simulink model "Lab1_mdl"  (R2013b)
settings: Solver=ode3  StartTime=0.0  StopTime=100.0  FixedStep=10e-3  RelTol=1e-3
undefined symbols (not defined in the file or in its folder): A, B, C
settings Model: Creator=user  LastModifiedBy=user
settings DataIOCC: LimitDataPoints=off

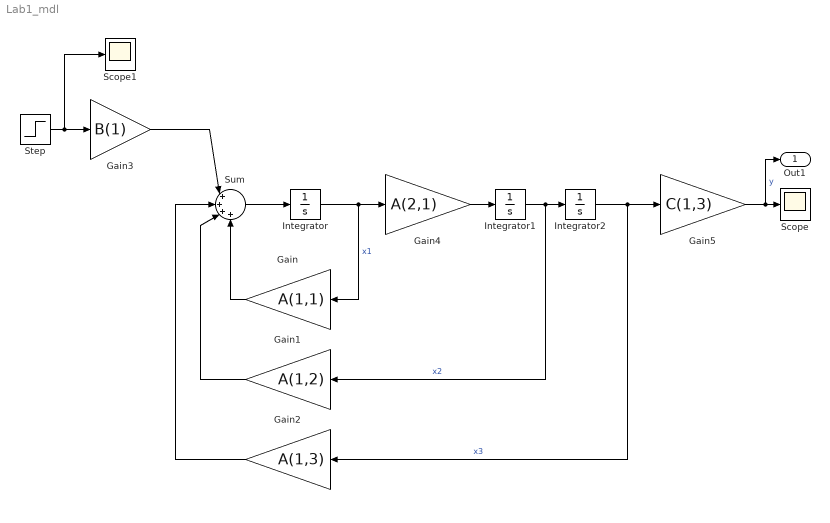
== system Lab1_mdl ==
  Gain : Gain  Gain=A(1,1)
  Gain1 : Gain  Gain=A(1,2)
  Gain2 : Gain  Gain=A(1,3)
  Gain3 : Gain  Gain=B(1)
  Gain4 : Gain  Gain=A(2,1)
  Gain5 : Gain  Gain=C(1,3)
  Integrator : Integrator
  Integrator1 : Integrator
  Integrator2 : Integrator
  Scope : Scope
      settings: SaveName=ContMdl_out
  Scope1 : Scope
      settings: SaveName=SetPoint
  Step : Step  Time=0  SampleTime=0
  Sum : Sum  Inputs=|++++
  Out1 : Outport
  wires:
  Sum/1 -> Integrator/1
  Gain/1 -> Sum/4
  Gain4/1 -> Integrator1/1
  Gain1/1 -> Sum/3
  Gain2/1 -> Sum/2
  Gain3/1 -> Sum/1
  Gain5/1 -> Out1/1, Scope/1  "y"
  Integrator/1 -> Gain4/1, Gain/1  "x1"
  Integrator1/1 -> Integrator2/1, Gain1/1  "x2"
  Integrator2/1 -> Gain5/1, Gain2/1  "x3"
  Step/1 -> Scope1/1, Gain3/1
